simulink model "cw7_model_BORKOWSKI_17"  (R2017b)
settings: Solver=VariableStepAuto  StartTime=0.0  StopTime=300  MaxStep=0.01  MinStep=0.001  RelTol=1e-6
values from neighbouring files (symbols this model uses):
  a0 = 1/(R1 *C1)    (= 0.1)    [cw7_dane_BORKOWSKI.m]
  a1 = 1/(R1*C2)    (= 0.2)    [cw7_dane_BORKOWSKI.m]
  a2 = 1/(R2*C2)    (= 0.1)    [cw7_dane_BORKOWSKI.m]
  b1 = 1/C1    (= 0.1)    [cw7_dane_BORKOWSKI.m]
  e = 0.1 * p0    (= 0.2)    [cw7_dane_BORKOWSKI.m]
  p0 = 2    [cw7_dane_BORKOWSKI.m]
  x10 = 3    [cw7_dane_BORKOWSKI.m]
  x20 = 2    [cw7_dane_BORKOWSKI.m]
settings Model: Creator=Student  LastModifiedBy=Student
settings DataIOCC: SaveFormat=Array
settings DebuggingCC: UnconnectedInputMsg=none  UnconnectedOutputMsg=none  UnconnectedLineMsg=none
settings ModelReferenceCC: EnableRefExpFcnMdlSchedulingChecks=off
settings SFSimCC: SimUseLocalCustomCode=on
settings RTWCC: Description=Generic Real-Time Target  RTWUseLocalCustomCode=on

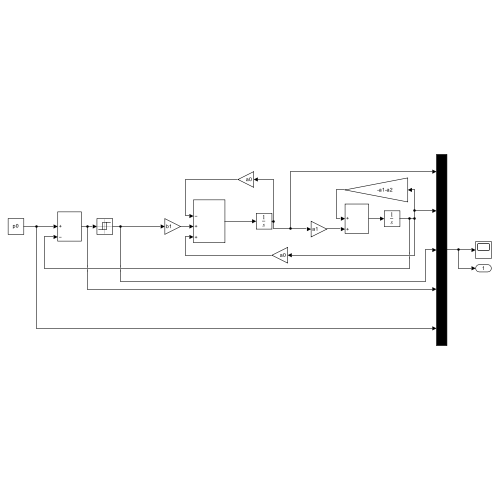
[thumbnail: Simulink's stored preview of the top-level diagram]
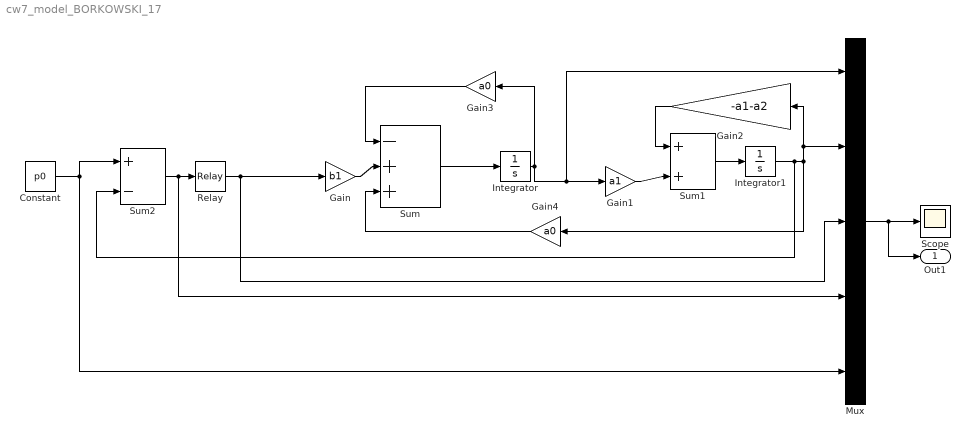
== system cw7_model_BORKOWSKI_17 ==
  Constant : Constant  Value=p0
  Gain : Gain  Gain=b1
  Gain1 : Gain  Gain=a1
  Gain2 : Gain  Gain=-a1-a2
  Gain3 : Gain  Gain=a0
  Gain4 : Gain  Gain=a0
  Integrator : Integrator  InitialCondition=x10
  Integrator1 : Integrator  InitialCondition=x20
  Mux : Mux  Inputs=5
  Relay : Relay  OnSwitchValue=e  OffSwitchValue=-e  OnOutputValue=u
  Scope : Scope
  Sum : Sum  Inputs=|-++
  Sum1 : Sum  Inputs=|++
  Sum2 : Sum  Inputs=|+-
  Out1 : Outport
  wires:
  Relay/1 -> Mux/3, Gain/1
  Integrator/1 -> Mux/1, Gain1/1, Gain3/1
  Gain/1 -> Sum/2
  Sum/1 -> Integrator/1
  Gain1/1 -> Sum1/2
  Gain3/1 -> Sum/1
  Sum1/1 -> Integrator1/1
  Integrator1/1 -> Sum2/2, Mux/2, Gain2/1, Gain4/1
  Gain2/1 -> Sum1/1
  Mux/1 -> Scope/1, Out1/1
  Gain4/1 -> Sum/3
  Constant/1 -> Mux/5, Sum2/1
  Sum2/1 -> Mux/4, Relay/1
